simulink model "KITTRacing"  (R2015b)
settings: Solver=FixedStepAuto  StartTime=0.0  StopTime=8  FixedStep=0.01  RelTol=1e-3
values from neighbouring files (symbols this model uses):
  b = 0.0015    [KITTParameters.m]
  c = 0.02    [KITTParameters.m]    (also in directionkeys.m = 0)
  Fa = 60    [KITTParameters.m]
  Fb = -120    [KITTParameters.m]
  m = 13    [KITTParameters.m]
  Vini = 0    [KITTParameters.m]
  xbrake = Xa    [KITTBrake.m]
undefined symbols (not defined in the file or in its folder): magnitude
libraries: simulink x2
settings Model: Creator=koenm  LastModifiedBy=koenm
settings DataIOCC: SaveFormat=StructureWithTime
settings DebuggingCC: AlgebraicLoopMsg=none

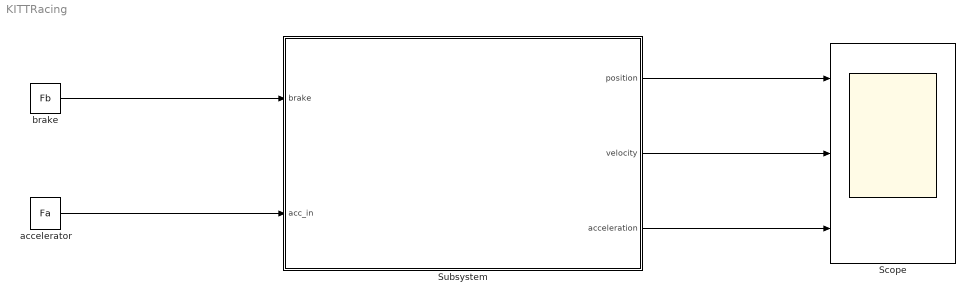
== system KITTRacing ==
  Scope : Scope  NumInputPorts=3
  Subsystem : Subsystem
  accelerator : Constant  Value=Fa
  brake : Constant  Value=Fb
  wires:
  brake/1 -> Subsystem/1(brake)
  accelerator/1 -> Subsystem/2(acc_in)
  Subsystem/1("position ") -> Scope/1
  Subsystem/2(velocity) -> Scope/2
  Subsystem/3(acceleration) -> Scope/3

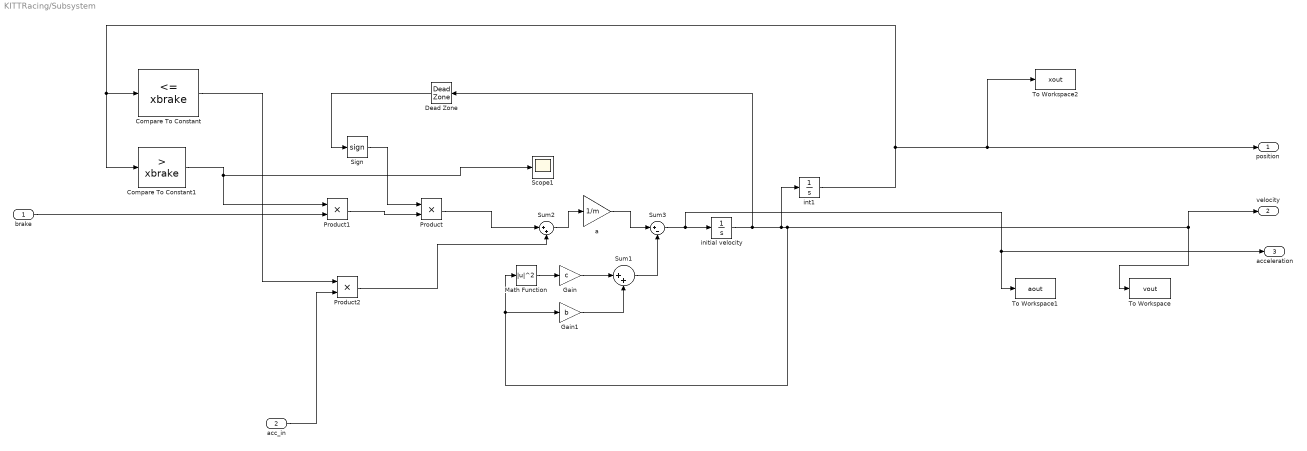
== system KITTRacing/Subsystem ==
  brake : Inport
  acc_in : Inport  Port=2
  Compare To Constant : simulink/Logic and Bit Operations/Compare To Constant  relop=<=  const=xbrake  OutDataTypeStr=boolean
  Compare To Constant1 : simulink/Logic and Bit Operations/Compare To Constant  relop=>  const=xbrake  OutDataTypeStr=boolean
  Dead Zone : DeadZone  LowerValue=-0.03  UpperValue=0.03  SaturateOnIntegerOverflow=on
  Gain : Gain  Gain=c
  Gain1 : Gain  Gain=b
  Math Function : Math  Operator=magnitude^2  SaturateOnIntegerOverflow=on
  Product : Product
  Product1 : Product
  Product2 : Product
  Scope1 : Scope
  Sign : Signum
  Sum1 : Sum  Inputs=|++
  Sum2 : Sum  Inputs=|++
  Sum3 : Sum  Inputs=|+-
  To Workspace : ToWorkspace  VariableName=vout  SaveFormat=Timeseries  SampleTime=-1
  To Workspace1 : ToWorkspace  VariableName=aout  SaveFormat=Timeseries  SampleTime=-1
  To Workspace2 : ToWorkspace  VariableName=xout  SaveFormat=Timeseries  SampleTime=-1
  a : Gain  Gain=1/m
  initial velocity : Integrator  InitialCondition=Vini
  int1 : Integrator
  "position " : Outport
  velocity : Outport  Port=2
  acceleration : Outport  Port=3
  wires:
  Gain/1 -> Sum1/1
  Gain1/1 -> Sum1/2
  Math Function/1 -> Gain/1
  Dead Zone/1 -> Sign/1
  Sign/1 -> Product/1
  int1/1 -> To Workspace2/1, "position "/1, Compare To Constant/1, Compare To Constant1/1
  initial velocity/1 -> Dead Zone/1, int1/1, To Workspace/1, velocity/1, Gain1/1, Math Function/1
  Sum2/1 -> a/1
  Product/1 -> Sum2/1
  acc_in/1 -> Product2/2
  Product2/1 -> Sum2/2
  brake/1 -> Product1/2
  Product1/1 -> Product/2
  Compare To Constant/1 -> Product2/1
  Compare To Constant1/1 -> Scope1/1, Product1/1
  Sum3/1 -> To Workspace1/1, acceleration/1, initial velocity/1
  Sum1/1 -> Sum3/2
  a/1 -> Sum3/1
